simulink model "PitchANDPlunge"  (R2018a)
settings: Solver=VariableStepAuto  StartTime=0.0  StopTime=100  FixedStep=0.0001  MaxStep=1e-2  RelTol=1e-3  EnableMultiTasking=on
values from neighbouring files (symbols this model uses):
  A = [-0.313 56.7 0; -0.0139 -0.426 0; 0 56.7 0]    [CoSim.m]
  B = [0.232; 0.0203; 0.0]    [CoSim.m]
  C = (y_hat-y_ref)'*(y_hat-y_ref)/length(y_hat)    [CoSim.m]
  ks = K(4)    [CoSim.m]
  pi1 = K(2)*1i    [CoSim.m]
  pr1 = K(1)    [CoSim.m]
  zr = K(3)    [CoSim.m]
undefined symbols (not defined in the file or in its folder): Kc, Td, Ti
libraries: simulink x4, slident x1, cstblocks x1
settings Model: Creator=rromano  LastModifiedBy=Felipe
settings SolverCC: ZeroCrossAlgorithm=Adaptive  AutoInsertRateTranBlk=on
settings DataIOCC: LimitDataPoints=on  SaveFormat=Array  SignalLoggingSaveFormat=ModelDataLogs
settings OptimizationCC: ExpressionDepthLimit=2147483647  LifeSpan=inf
settings DebuggingCC: AlgebraicLoopMsg=none  UnderspecifiedInitializationDetection=Classic  MergeDetectMultiDrivingBlocksExec=none  MaxConsecutiveZCsMsg=none  SolverPrmCheckMsg=warning  FcnCallInpInsideContextMsg=warning  StateNameClashWarn=warning  SFUnexpectedBacktrackingDiag=warning  SFNoUnconditionalDefaultTransitionDiag=warning  SFExecutionAtInitializationDiag=none
settings HardwareCC: ProdBitPerPointer=32  ProdBitPerSizeT=32  ProdBitPerPtrDiffT=32  ProdLargestAtomicFloat=None  ProdIntDivRoundTo=Undefined  ProdEndianess=Unspecified  ProdWordSize=32  ProdHWDeviceType=32-bit Generic
settings ModelReferenceCC: PropagateSignalLabelsOutOfModel=off
settings CodeAppCC: StateflowObjectComments=on
settings GRTTargetCC: TargetLangStandard=C89/C90 (ANSI)  GeneratePreprocessorConditionals=Disable all  CombineOutputUpdateFcns=off  GRTInterface=on
settings ConfigComp: CovMetricSettings=dw  CovHtmlReporting=on  CovSaveCumulativeToWorkspaceVar=on  CovSaveSingleToWorkspaceVar=on  CovExternalEMLEnable=off

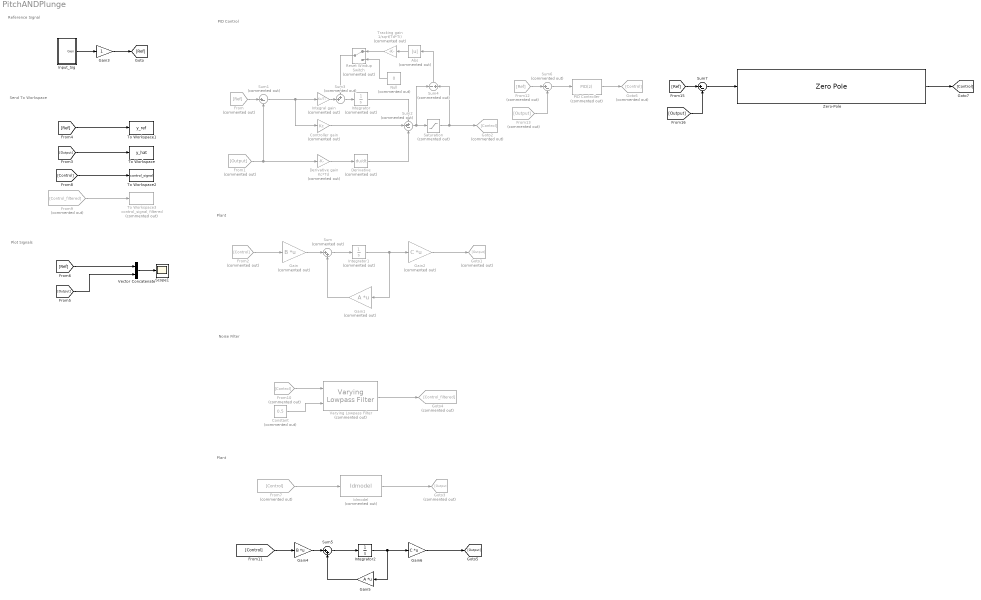
== system PitchANDPlunge ==
  note: Noise Filter
  note: Plot Signals
  note: Send To Workspace
  note: Reference Signal
  note: PID Control
  note: Plant
  note: Plant
  Abs : Abs  Commented=on
  Constant : Constant  Commented=on  Value=0.5
  Controller gain : Gain  Commented=on  Gain=Kc
  Derivative : Derivative  Commented=on
  Derivative gain : Gain  Commented=on  Gain=Kc*Td
  From : From  Commented=on  GotoTag=Ref
  From1 : From  Commented=on  GotoTag=Output
  From10 : From  Commented=on  GotoTag=Control
  From12 : From  Commented=on  GotoTag=Ref
  From13 : From  Commented=on  GotoTag=Output
  From2 : From  Commented=on  GotoTag=Control
  From7 : From  Commented=on  GotoTag=Control
  From9 : From  Commented=on  GotoTag=Control_filtered
  Gain : Gain  Commented=on  Gain=B  Multiplication=Matrix(K*u)
  Gain1 : Gain  Commented=on  Gain=A  Multiplication=Matrix(K*u)
  Gain2 : Gain  Commented=on  Gain=C  Multiplication=Matrix(K*u)
  Gain3 : Gain
  Gain4 : Gain  Gain=B  Multiplication=Matrix(K*u)
  Gain5 : Gain  Gain=A  Multiplication=Matrix(K*u)
  Gain6 : Gain  Gain=C  Multiplication=Matrix(K*u)
  Goto1 : Goto  Commented=on  GotoTag=Output
  Goto2 : Goto  Commented=on  GotoTag=Control
  Goto3 : Goto  Commented=on  GotoTag=Output
  Goto4 : Goto  Commented=on  GotoTag=Control_filtered
  Goto6 : Goto  Commented=on  GotoTag=Control
  Idmodel : slident/Models/Idmodel  Commented=on  sys=Continuos_model  IC=0  noi=off  seed=[]
      settings: SourceProductName=System Identification Toolbox  SourceProductBaseCode=ID
  Input_Sig : Subsystem
  Integral gain : Gain  Commented=on  Gain=Kc/Ti
  Integrator : Integrator  Commented=on  ZeroCross=off
  Integrator1 : Integrator  Commented=on
  Integrator2 : Integrator  ZeroCross=off
  Null : Constant  Commented=on  Value=0
  PID Controller : simulink/Continuous/PID Controller  Commented=on  Controller=PID  TimeDomain=Discrete-time  SampleTime=-1  IntegratorMethod=Forward Euler  FilterMethod=Forward Euler  Form=Parallel  UseFilter=on  ControllerParametersSource=internal  P=Kc  I=Ti  D=Td  N=100  InitialConditionSource=internal  InitialConditionForIntegrator=0  InitialConditionForFilter=0  ExternalReset=none  LimitOutput=on  UpperSaturationLimit=24  LowerSaturationLimit=-24  LinearizeAsGain=on  AntiWindupMode=none  Kb=1  TrackingMode=off  Kt=1  PParamMin=[]  PParamMax=[]  IParamMin=[]  IParamMax=[]  DParamMin=[]  DParamMax=[]  NParamMin=[]  NParamMax=[]  KbParamMin=[]  KbParamMax=[]  KtParamMin=[]  KtParamMax=[]  POutMin=[]  POutMax=[]  IOutMin=[]  IOutMax=[]  DOutMin=[]  DOutMax=[]  NOutMin=[]  NOutMax=[]  KbOutMin=[]  KbOutMax=[]  KtOutMin=[]  KtOutMax=[]  IntegratorOutMin=[]  IntegratorOutMax=[]  FilterOutMin=[]  FilterOutMax=[]  SumOutMin=[]  SumOutMax=[]  SumI1OutMin=[]  SumI1OutMax=[]  SumI2OutMin=[]  SumI2OutMax=[]  SumI3OutMin=[]  SumI3OutMax=[]  SumDOutMin=[]  SumDOutMax=[]  SaturationOutMin=[]  SaturationOutMax=[]  IntegratorContinuousStateAttributes=''  IntegratorStateMustResolveToSignalObject=off  IntegratorRTWStateStorageClass=Auto  FilterContinuousStateAttributes=''  FilterStateMustResolveToSignalObject=off  FilterRTWStateStorageClass=Auto  DifferentiatorICPrevScaledInput=0  DifferentiatorOutMin=[]  DifferentiatorOutMax=[]  FilterDiffOutCoefMin=[]  FilterDiffOutCoefMax=[]  SumDenOutMin=[]  SumDenOutMax=[]  SumNumOutMin=[]  SumNumOutMax=[]  ReciprocalOutMin=[]  ReciprocalOutMax=[]  DivideOutMin=[]  DivideOutMax=[]  TunerSelectOption=Transfer Function Based (PID Tuner App)
  Reset Windup Switch : ManualSwitch  Commented=on
  Saturation : Saturate  Commented=on  UpperLimit=12  LowerLimit=-12  ZeroCross=off
  Scope1 : Scope
  Sum : Sum  Commented=on  Inputs=|++
  Sum1 : Sum  Commented=on  Inputs=|+-
  Sum2 : Sum  Commented=on  Inputs=++-
  Sum3 : Sum  Commented=on  Inputs=++|
  Sum4 : Sum  Commented=on  Inputs=-|+
  Sum5 : Sum  Inputs=|++
  Sum6 : Sum  Commented=on  Inputs=|+-
  Sum7 : Sum  Inputs=|+-
  To Workspace : ToWorkspace  VariableName=y_hat  SampleTime=-1
      settings: Save2DSignal=2-D array (concatenate along first dimension)
  To Workspace1 : ToWorkspace  VariableName=y_ref  SampleTime=-1
      settings: Save2DSignal=2-D array (concatenate along first dimension)
  To Workspace2 : ToWorkspace  VariableName=control_signal  SampleTime=-1
      settings: Save2DSignal=2-D array (concatenate along first dimension)
  To Workspace3 : ToWorkspace  Commented=on  VariableName=control_signal_filtered  SaveFormat=Timeseries  SampleTime=-1
      settings: Save2DSignal=2-D array (concatenate along first dimension)
  Tracking gain : Gain  Commented=on  Gain=1/sqrt(Td*Ti)
  Varying Lowpass Filter : cstblocks/Linear Parameter Varying/Varying Lowpass Filter  Commented=on  N=1
      settings: SourceProductName=Control System Toolbox
  Vector Concatenate : Concatenate
  Zero-Pole : ZeroPole  Zeros=[-zr]  Poles=[0 -pr1+pi1 -pr1-pi1]  Gain=[ks]
  wires:
  Vector Concatenate/1 -> Scope1/1
  Input_Sig/1(Gen) -> Gain3/1
  Reset Windup Switch/1 -> Sum3/1
  Tracking gain/1 -> Reset Windup Switch/1
  Null/1 -> Reset Windup Switch/2
  Derivative/1 -> Sum2/3
  Controller gain/1 -> Sum2/2
  Derivative gain/1 -> Derivative/1
  Sum3/1 -> Integrator/1
  Saturation/1 -> Goto2/1, Sum4/2
  Sum2/1 -> Sum4/1, Saturation/1
  Integrator/1 -> Sum2/1
  Integral gain/1 -> Sum3/2
  Gain/1 -> Sum/1
  Sum/1 -> Integrator1/1
  Gain1/1 -> Sum/2
  Integrator1/1 -> Gain2/1, Gain1/1
  From/1 -> Sum1/1
  Sum1/1 -> Controller gain/1, Integral gain/1
  Gain2/1 -> Goto1/1
  From2/1 -> Gain/1
  [Output] -> To Workspace/1
  [Ref] -> To Workspace1/1
  [Ref] -> Vector Concatenate/1
  [Output] -> Vector Concatenate/2
  Idmodel/1 -> Goto3/1
  From7/1 -> Idmodel/1
  From1/1 -> Derivative gain/1, Sum1/2
  [Control] -> To Workspace2/1
  From9/1 -> To Workspace3/1
  From10/1 -> Varying Lowpass Filter/1
  Constant/1 -> Varying Lowpass Filter/2
  Varying Lowpass Filter/1 -> Goto4/1
  Gain3/1 -> [Ref]
  Gain6/1 -> [Output]
  [Control] -> Gain4/1
  Gain4/1 -> Sum5/1
  Sum5/1 -> Integrator2/1
  Gain5/1 -> Sum5/2
  Integrator2/1 -> Gain5/1, Gain6/1
  Abs/1 -> Tracking gain/1
  Sum4/1 -> Abs/1
  From12/1 -> Sum6/1
  From13/1 -> Sum6/2
  Sum6/1 -> PID Controller/1
  PID Controller/1 -> Goto6/1
  [Ref] -> Sum7/1
  [Output] -> Sum7/2
  Sum7/1 -> Zero-Pole/1
  Zero-Pole/1 -> [Control]

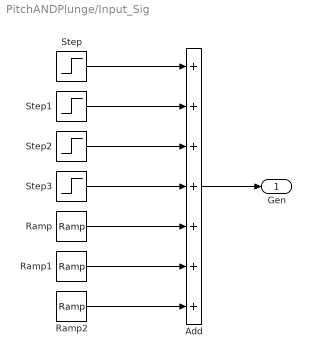
== system PitchANDPlunge/Input_Sig ==
  Add : Sum  Inputs=+++++++
  Ramp : simulink/Sources/Ramp  slope=2  start=70  InitialOutput=0
  Ramp1 : simulink/Sources/Ramp  slope=-4  start=80  InitialOutput=0
  Ramp2 : simulink/Sources/Ramp  slope=2  start=90  InitialOutput=0
  Step : Step  Time=5  After=10  SampleTime=0
  Step1 : Step  Time=25  After=-20  SampleTime=0
  Step2 : Step  Time=35  After=35  SampleTime=0
  Step3 : Step  Time=50  After=-25  SampleTime=0
  Gen : Outport
  wires:
  Ramp1/1 -> Add/6
  Ramp2/1 -> Add/7
  Step3/1 -> Add/4
  Step2/1 -> Add/3
  Ramp/1 -> Add/5
  Add/1 -> Gen/1
  Step1/1 -> Add/2
  Step/1 -> Add/1
